simulink model "inport_outport"  (R2021a)
settings: Solver=VariableStepAuto  StartTime=0.0  StopTime=1.0  RelTol=1e-3
libraries: dspswit3 x1, dspsigops x1
settings Model: Creator=Acer  LastModifiedBy=Acer
settings DataIOCC: LoadExternalInput=on

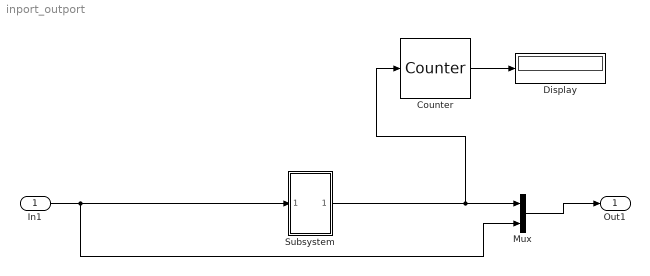
== system inport_outport ==
  In1 : Inport
  Counter : dspswit3/Counter  Direction=Up  CountEvent=Rising edge  CounterSize=8 bits  MaxCount=255  InitialCount=0  Output=Count  HitValue=32  ResetInput=off  SamplesPerFrame=1  Ts=1  CntDtype=double  HitDtype=Logical
  Display : Display
  Mux : Mux  Inputs=2
  Subsystem : Subsystem
  Out1 : Outport
  wires:
  In1/1 -> Subsystem/1(In1), Mux/2
  Counter/1 -> Display/1
  Mux/1 -> Out1/1
  Subsystem/1(Out1) -> Counter/1, Mux/1

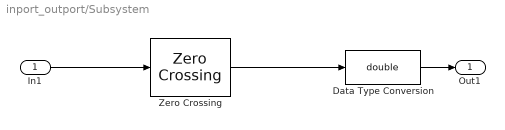
== system inport_outport/Subsystem ==
  In1 : Inport
  Data Type Conversion : DataTypeConversion  OutDataTypeStr=double
  Zero Crossing : dspsigops/Zero Crossing  InputProcessing=Columns as channels (frame based)
      settings: SourceProductBaseCode=DS
  Out1 : Outport
  wires:
  Zero Crossing/1 -> Data Type Conversion/1
  In1/1 -> Zero Crossing/1
  Data Type Conversion/1 -> Out1/1
